simulink model "pendulum"  (R2021a)
settings: Solver=VariableStepAuto  StartTime=0.0  StopTime=50  FixedStep=ts  RelTol=1e-3  AbsTol=1e-3  EnableMultiTasking=on
undefined symbols (not defined in the file): kd, kp, l, m, ts_algo
libraries: sm_lib x4, nesl_utility x4, simulink_extras x2
settings Model: Creator=Maxim  LastModifiedBy=Maxim
settings SolverCC: AutoScaleAbsTol=off  AlgebraicLoopSolver=TrustRegion
settings DataIOCC: LimitDataPoints=on  MaxDataPoints=10000
settings OptimizationCC: LifeSpan=inf
settings DebuggingCC: AllowSymbolicDim=off  SFUnexpectedBacktrackingDiag=warning  SFNoUnconditionalDefaultTransitionDiag=warning  SFExecutionAtInitializationDiag=none  SFMachineParentedDataDiag=warning  ArithmeticOperatorsInVariantConditions=warning
settings SFSimCC: SimUseLocalCustomCode=off  CustomCodeUndefinedFunction=UseInterfaceOnly
settings RTWCC: RTWUseLocalCustomCode=off
settings CodeAppCC: StateflowObjectComments=on
settings GRTTargetCC: TargetLangStandard=C89/C90 (ANSI)
settings ConfigComp: CovMetricSettings=dw  CovSaveCumulativeToWorkspaceVar=on  CovSaveSingleToWorkspaceVar=on  CovExternalEMLEnable=off  CovSFcnEnable=off
settings SimscapeCC: SimscapeLogType=all  SimscapeLogSimulationStatistics=on  SimscapeLogDataHistory=10000

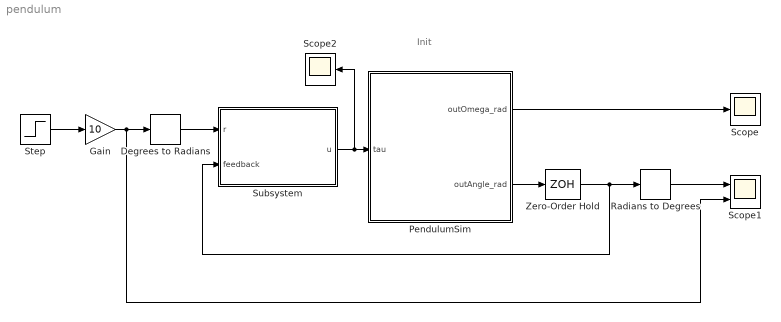
== system pendulum ==
  note: Init
  Degrees to Radians : simulink_extras/Transformations/Degrees to Radians
  Gain : Gain  Gain=10
  PendulumSim : Subsystem
  Radians to Degrees : simulink_extras/Transformations/Radians to Degrees
  Scope : Scope
  Scope1 : Scope  NumInputPorts=2
  Scope2 : Scope
  Step : Step  Time=0  SampleTime=ts_algo
  Subsystem : Subsystem
  Zero-Order Hold : ZeroOrderHold  SampleTime=ts_algo
  wires:
  PendulumSim/1(outOmega_rad) -> Scope/1
  PendulumSim/2(outAngle_rad) -> Zero-Order Hold/1
  Zero-Order Hold/1 -> Radians to Degrees/1, Subsystem/2(feedback)
  Subsystem/1(u) -> Scope2/1, PendulumSim/1(tau)
  Radians to Degrees/1 -> Scope1/1
  Gain/1 -> Scope1/2, Degrees to Radians/1
  Step/1 -> Gain/1
  Degrees to Radians/1 -> Subsystem/1(r)

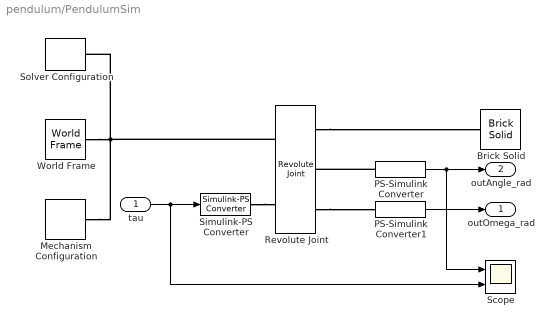
== system pendulum/PendulumSim ==
  tau : Inport
  Brick Solid : sm_lib/Body Elements/Brick Solid  GraphicAmbientColor=[0.15 0.15 0.15 1.0]  BasedOnType=Density  BrickDimensions=[0.01 0.1 0.01]  BrickDimensionUnits=m  CenterOfMass=[0 0 0]  CenterOfMassUnits=m  GraphicDiffuseColor=[1.0 0.2 0.2]  Density=100000  DensityUnits=kg/m^3  DoExposeReferenceFrame=on  GraphicEmissiveColor=[0.0 0.0 0.0 1.0]  ExportEntireGeometry=off  SerializedFrames=<Frames><Frame><Id>Frame1</Id><Value><Name>F1</Name><Origin><Source>GeometricFeature</Source><FeatureName>-y surface</FeatureName></Origin><PrimaryAxis><DefinedDirection>+Z</DefinedDirection><Source>ReferenceFrame</Source><SourceDirection>+Z</SourceDirection><FeatureName></FeatureName></PrimaryAxis><SecondaryAxis><DefinedDirection>+X</DefinedDirection><Source>ReferenceFrame</Source><SourceDirection>+X</SourceDirection><FeatureName></FeatureName></SecondaryAxis></Value></Frame></Frames>  MarkerShape=Sphere  MarkerSize=10  GraphicType=FromGeometry  InertiaType=CalculateFromGeometry  Mass=1  MassUnits=kg  MomentsOfInertia=[1 1 1]  MomentsOfInertiaUnits=kg*m^2  GraphicOpacity=1.0  ProductsOfInertia=[0 0 0]  ProductsOfInertiaUnits=kg*m^2  GraphicShininess=75  GraphicSpecularColor=[0.5 0.5 0.5 1.0]  GraphicVisPropType=SimpleVisualProperties
  Mechanism Configuration : sm_lib/Utilities/Mechanism Configuration  UniformGravity=Constant  GravityVector=[0 -9.80665 0]  GravityVectorUnits=m/s^2  GravityUnits=m/s^2  LinearizationDelta=0.001  JointModeTransitionNonlinearIterations=2
  PS-Simulink Converter : nesl_utility/PS-Simulink Converter  PhysicalDomain=network_engine_domain  SubClassName=ps_output  LeftPortType=input  RightPortType=output  PseudoPeriodic=off  Frequencies=[]  Unit=inherit  AffineConversion=off
      settings: SourceProductBaseCode=PW,SS
  PS-Simulink Converter1 : nesl_utility/PS-Simulink Converter  PhysicalDomain=network_engine_domain  SubClassName=ps_output  LeftPortType=input  RightPortType=output  PseudoPeriodic=off  Frequencies=[]  Unit=inherit  AffineConversion=off
      settings: SourceProductBaseCode=PW,SS
  Revolute Joint : sm_lib/Joints/Revolute Joint  JointMode=Normal  SenseConstraintForce=off  SenseConstraintForceX=off  SenseConstraintForceY=off  SenseConstraintForceZ=off  SenseConstraintTorque=off  SenseConstraintTorqueX=off  SenseConstraintTorqueY=off  SenseConstraintTorqueZ=off  SenseTotalForce=off  SenseTotalForceX=off  SenseTotalForceY=off  SenseTotalForceZ=off  SenseTotalTorque=off  SenseTotalTorqueX=off  SenseTotalTorqueY=off  SenseTotalTorqueZ=off  CompositeWrenchDir=FollowerOnBase  CompositeWrenchFrame=BaseFrame  EquilibriumPosition=0  EquilibriumPositionUnits=deg  SpringStiffness=0  SpringStiffnessUnits=N*m/deg  DampingCoefficient=0.1  DampingCoefficientUnits=N*m/(deg/s)  TorqueActuationMode=InputTorque  MotionActuationMode=ComputedMotion  SensePosition=on  SenseVelocity=on  SenseAcceleration=off  SenseTorqueForce=off  SenseLowerLimitTorqueForce=off  SenseUpperLimitTorqueForce=off  LowerLimitSpecify=off  LowerLimitBound=-90  LowerLimitBoundUnits=deg  LowerLimitStiffness=1e4  LowerLimitStiffnessUnits=N*m/deg  LowerLimitDamping=10  LowerLimitDampingUnits=N*m/(deg/s)  LowerLimitTransitionRegionWidth=0.1  LowerLimitTransitionRegionWidthUnits=deg  UpperLimitSpecify=off  UpperLimitBound=90  UpperLimitBoundUnits=deg  UpperLimitStiffness=1e4  UpperLimitStiffnessUnits=N*m/deg  UpperLimitDamping=10  UpperLimitDampingUnits=N*m/(deg/s)  UpperLimitTransitionRegionWidth=0.1  UpperLimitTransitionRegionWidthUnits=deg  PositionTargetSpecify=off  PositionTargetPriority=High  PositionTargetValue=0  PositionTargetValueUnits=deg  VelocityTargetSpecify=off  VelocityTargetPriority=High  VelocityTargetValue=0  VelocityTargetValueUnits=deg/s
  Scope : Scope  NumInputPorts=2
  Simulink-PS Converter : nesl_utility/Simulink-PS Converter  PhysicalDomain=network_engine_domain  SubClassName=ps_input  LeftPortType=input  RightPortType=output  PseudoPeriodic=off  Frequencies=[]  NoiseDistribution=none  NoiseParameters=[]  Unit=1  AffineConversion=off  FilteringAndDerivatives=provide  SimscapeFilterOrder=1  InputFilterTimeConstant=0.001  UdotUserProvided=0
      settings: SourceProductBaseCode=PW,SS
  Solver Configuration : nesl_utility/Solver Configuration  PhysicalDomain=network_engine_domain  SubClassName=solver  LeftPortType=input  RightPortType=generic  Tones=[]  Harmonics=[]  SimulateNoise=off  Profile=off  UseLocalSampling=off  EnableSwitchedLinearOptims=on  FrequencyDomain=off  UseCCode=off  RelTol=0.001  AbsTol=1e-06  MinStep=1e-09  ToWorkspace=off  RevertToSquareIcSolve=off  NumHomotopyIterations=100  PhasorMode=off  PhasorModeNumHarmonics=1  DoDC=off  ResidualTolerance=1e-09  UseLocalSolver=off  LocalSolverChoice=NE_BACKWARD_EULER_ADVANCER  LocalSolverSampleTime=0.001  DoFixedCost=off  MaxNonlinIter=3  MaxModeIter=2  ComputeImpulses=off  ImpulseIterations=2  LinearAlgebra=Sparse  EquationFormulation=NE_TIME_EF  DelaysMemoryBudget=1024  AutomaticFiltering=on  FilteringTimeConstant=0.001  PartitionStorageMethod=AS_NEEDED  PartitionMemoryBudget=1024  PartitionMethod=FAST
      settings: SourceProductBaseCode=PW,SS
  World Frame : sm_lib/Frames and Transforms/World Frame
  outOmega_rad : Outport
  outAngle_rad : Outport  Port=2
  wires:
  tau/1 -> Scope/2, Simulink-PS Converter/1
  PS-Simulink Converter/1 -> Scope/1, outAngle_rad/1
  PS-Simulink Converter1/1 -> outOmega_rad/1
  connections:
  PS-Simulink Converter/LConn1 -- Revolute Joint/RConn2
  World Frame/RConn1 -- Solver Configuration/RConn1 -- Revolute Joint/LConn1 -- Mechanism Configuration/RConn1
  Simulink-PS Converter/RConn1 -- Revolute Joint/LConn2
  Revolute Joint/RConn3 -- PS-Simulink Converter1/LConn1
  Revolute Joint/RConn1 -- Brick Solid/LConn1

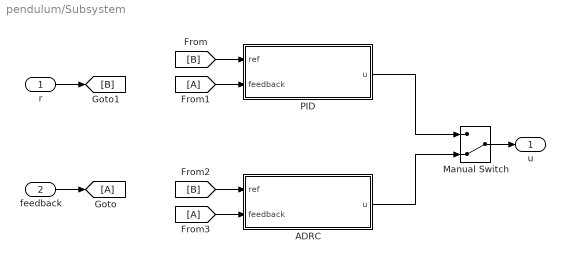
== system pendulum/Subsystem ==
  r : Inport
  feedback : Inport  Port=2
  ADRC : Subsystem
  Manual Switch : ManualSwitch  CurrentSetting=0
  PID : Subsystem
  u : Outport
  wires:
  r/1 -> [B]
  feedback/1 -> [A]
  [B] -> PID/1(ref)
  [A] -> PID/2(feedback)
  [B] -> ADRC/1(ref)
  [A] -> ADRC/2(feedback)
  Manual Switch/1 -> u/1
  PID/1(u) -> Manual Switch/1
  ADRC/1(u) -> Manual Switch/2

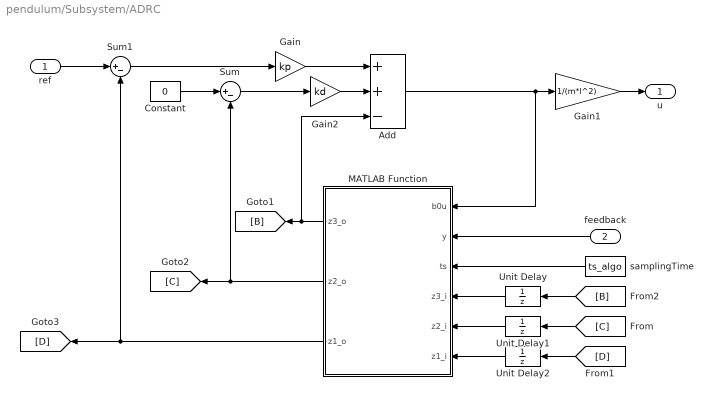
== system pendulum/Subsystem/ADRC ==
  ref : Inport
  feedback : Inport  Port=2
  Add : Sum  Inputs=++-
  Constant : Constant  Value=0
  Gain : Gain  Gain=kp
  Gain1 : Gain  Gain=1/(m*l^2)
  Gain2 : Gain  Gain=kd
  MATLAB Function : MATLAB Function  TreatAsAtomicUnit=on
  Sum : Sum  Inputs=|+-
  Sum1 : Sum  Inputs=|+-
  Unit Delay : UnitDelay  SampleTime=ts_algo  HasFrameUpgradeWarning=on
  Unit Delay1 : UnitDelay  SampleTime=ts_algo  HasFrameUpgradeWarning=on
  Unit Delay2 : UnitDelay  SampleTime=ts_algo  HasFrameUpgradeWarning=on
  samplingTime : Constant  Value=ts_algo
  u : Outport
  wires:
  Constant/1 -> Sum/1
  ref/1 -> Sum1/1
  Sum1/1 -> Gain/1
  Sum/1 -> Gain2/1
  Gain/1 -> Add/1
  Gain2/1 -> Add/2
  Gain1/1 -> u/1
  Add/1 -> MATLAB Function/1(b0u), Gain1/1
  MATLAB Function/1(z3_o) -> [B], Add/3
  MATLAB Function/2(z2_o) -> [C], Sum/2
  MATLAB Function/3(z1_o) -> [D], Sum1/2
  Unit Delay/1 -> MATLAB Function/4(z3_i)
  Unit Delay1/1 -> MATLAB Function/5(z2_i)
  Unit Delay2/1 -> MATLAB Function/6(z1_i)
  [C] -> Unit Delay1/1
  [D] -> Unit Delay2/1
  [B] -> Unit Delay/1
  samplingTime/1 -> MATLAB Function/3(ts)
  feedback/1 -> MATLAB Function/2(y)

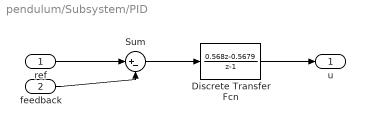
== system pendulum/Subsystem/PID ==
  ref : Inport
  feedback : Inport  Port=2
  Discrete Transfer Fcn : DiscreteTransferFcn  Numerator=[0.568 -0.5679]  Denominator=[1 -1]
  Sum : Sum  Inputs=|+-
  u : Outport
  wires:
  ref/1 -> Sum/1
  feedback/1 -> Sum/2
  Discrete Transfer Fcn/1 -> u/1
  Sum/1 -> Discrete Transfer Fcn/1

== matlab function pendulum/Subsystem/ADRC/MATLAB Function ==
  data: z3_o output; z2_o output; z1_o output; b0u input; y input; ts input; z3_i input; z2_i input; z1_i input
function [z3_o, z2_o, z1_o] = fcn(b0u, y, ts, z3_i, z2_i, z1_i)
% Estimation params
k1 = 1; k2 = 1; k3 = 1; 

% The update
e = z1_i-y;
z1_o = z1_i + ts*z2_i - k1*e;
z2_o = z2_i + ts*(z3_i+b0u) - k2*e;
z3_o = z3_i - k3*e;
